simulink model "sim_environment_gcc"  (Simulink 8.6)
settings: Solver=VariableStepAuto  StartTime=0.0  StopTime=100  RelTol=1e-3
values from neighbouring files (symbols this model uses):
  controller_parameters = struct()    [sim_init.m]
  simulation_parameters = struct()    [sim_init.m]
  vehicle_parameters = struct()    [sim_init.m]
libraries: aerolibactuator x3
settings Model: Creator=cmasserafilho  LastModifiedBy=cmasserafilho
settings DataIOCC: LimitDataPoints=off  SaveFormat=Dataset  SignalLoggingSaveFormat=Dataset  ReturnWorkspaceOutputs=on
settings OptimizationCC: ExpressionDepthLimit=128
settings DebuggingCC: UnderspecifiedInitializationDetection=Simplified  MergeDetectMultiDrivingBlocksExec=error  SolverPrmCheckMsg=none  FcnCallInpInsideContextMsg=EnableAllAsError  StateNameClashWarn=none
settings HardwareCC: ProdBitPerPointer=64  ProdLargestAtomicFloat=Float  ProdIntDivRoundTo=Zero  ProdEndianess=LittleEndian  ProdWordSize=64  ProdHWDeviceType=Intel->x86-64 (Windows64)
settings GRTTargetCC: GeneratePreprocessorConditionals=Use local settings  CombineOutputUpdateFcns=on  GRTInterface=off
settings ConfigComp: CovModelRefEnable=off

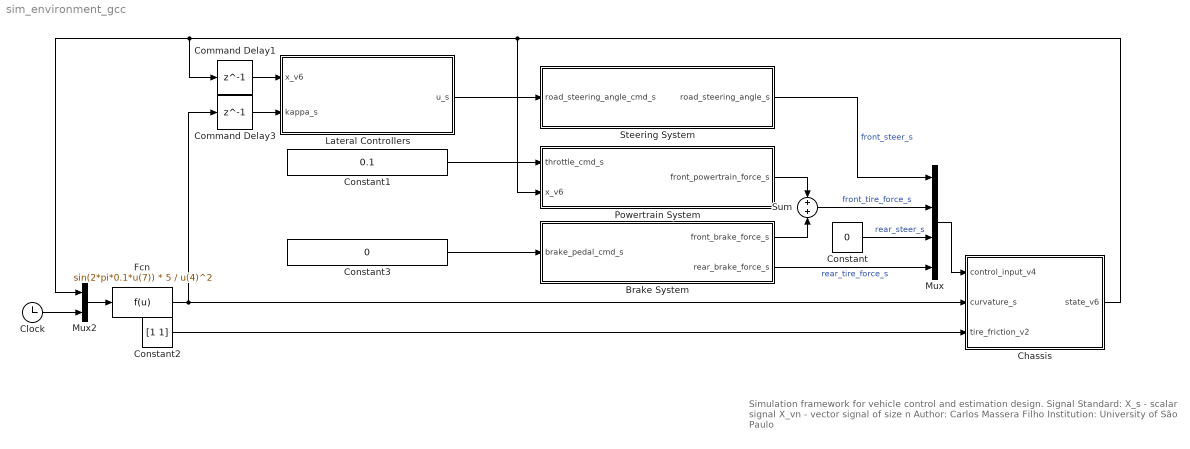
== system sim_environment_gcc ==
  note: Simulation framework for vehicle control and estimation design.
      |
      | Signal Standard:
      | X_s - scalar signal
      | X_vn - vector signal of size n
      |
      | Author: Carlos Massera Filho
      | Institution: University of São Paulo
  Brake System : Subsystem
  Chassis : Subsystem
  Clock : Clock
  Command Delay1 : Delay  DelayLength=1  InitialCondition=0  SampleTime=controller_parameters.Ts
  Command Delay3 : Delay  DelayLength=1  InitialCondition=0  SampleTime=controller_parameters.Ts
  Constant : Constant  Value=0
  Constant1 : Constant  Value=0.1  SampleTime=Inf
  Constant2 : Constant  Value=[1 1]
  Constant3 : Constant  Value=0
  Fcn : Fcn  Expr=sin(2*pi*0.1*u(7)) * 5 / u(4)^2
  Lateral Controllers : MATLAB Function  TreatAsAtomicUnit=on
  Mux : Mux
  Mux2 : Mux  Inputs=2
  Powertrain System : Subsystem
  Steering System : Subsystem
  Sum : Sum  Inputs=+|+
  wires:
  Chassis/1(state_v6) -> Command Delay1/1, Mux2/1, Powertrain System/2(x_v6)
  Mux/1 -> Chassis/1(control_input_v4)
  Constant/1 -> Mux/3  "rear_steer_s"
  Sum/1 -> Mux/2  "front_tire_force_s"
  Brake System/2(rear_brake_force_s) -> Mux/4  "rear_tire_force_s"
  Brake System/1(front_brake_force_s) -> Sum/2
  Powertrain System/1(front_powertrain_force_s) -> Sum/1
  Steering System/1("road_steering_angle_s ") -> Mux/1  "front_steer_s"
  Lateral Controllers/1(u_s) -> Steering System/1(road_steering_angle_cmd_s)
  Constant2/1 -> Chassis/3(tire_friction_v2)
  Command Delay1/1 -> Lateral Controllers/1(x_v6)
  Command Delay3/1 -> Lateral Controllers/2(kappa_s)
  Fcn/1 -> Command Delay3/1, Chassis/2(curvature_s)
  Mux2/1 -> Fcn/1
  Clock/1 -> Mux2/2
  Constant3/1 -> Brake System/1(brake_pedal_cmd_s)
  Constant1/1 -> Powertrain System/1(throttle_cmd_s)

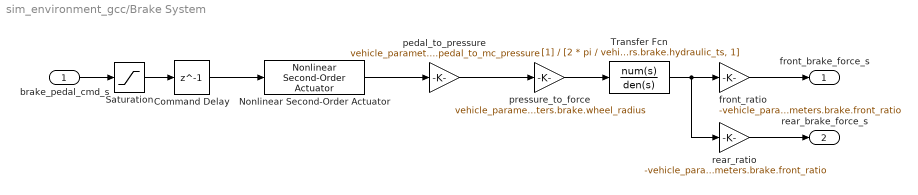
== system sim_environment_gcc/Brake System ==
  brake_pedal_cmd_s : Inport
  Command Delay : Delay  DelayLength=1  InitialCondition=0  SampleTime=vehicle_parameters.brake.delay
  Nonlinear Second-Order Actuator : aerolibactuator/Nonlinear Second-Order Actuator  wn_fin=2 * pi / vehicle_parameters.brake.actuator_tc  z_fin=1  fin_max=1  fin_min=0  fin_maxrate=vehicle_parameters.brake.rate_limit  fin_act_0=0  fin_act_vel=0
  Saturation : Saturate  UpperLimit=1  LowerLimit=0
  Transfer Fcn : TransferFcn  Denominator=[2 * pi / vehicle_parameters.brake.hydraulic_ts, 1]
  front_ratio : Gain  Gain=-vehicle_parameters.brake.front_ratio
  pedal_to_pressure : Gain  Gain=vehicle_parameters.brake.pedal_to_mc_pressure
  pressure_to_force : Gain  Gain=vehicle_parameters.brake.mc_pressure_to_torque / vehicle_parameters.brake.wheel_radius
  rear_ratio : Gain  Gain=-vehicle_parameters.brake.front_ratio
  front_brake_force_s : Outport
  rear_brake_force_s : Outport  Port=2
  wires:
  brake_pedal_cmd_s/1 -> Saturation/1
  front_ratio/1 -> front_brake_force_s/1
  rear_ratio/1 -> rear_brake_force_s/1
  Saturation/1 -> Command Delay/1
  Nonlinear Second-Order Actuator/1 -> pedal_to_pressure/1
  Command Delay/1 -> Nonlinear Second-Order Actuator/1
  pressure_to_force/1 -> Transfer Fcn/1
  Transfer Fcn/1 -> rear_ratio/1, front_ratio/1
  pedal_to_pressure/1 -> pressure_to_force/1

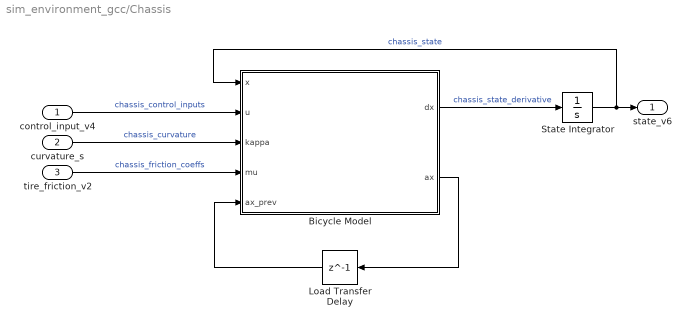
== system sim_environment_gcc/Chassis ==
  control_input_v4 : Inport
  curvature_s : Inport  Port=2
  tire_friction_v2 : Inport  Port=3
  Bicycle Model : MATLAB Function  TreatAsAtomicUnit=on
  Load Transfer Delay : Delay  DelayLength=1  InitialCondition=0  SampleTime=vehicle_parameters.uncertainty.load_transfer_Ts
  State Integrator : Integrator  InitialCondition=simulation_parameters.x0
  state_v6 : Outport
  wires:
  control_input_v4/1 -> Bicycle Model/2(u)  "chassis_control_inputs"
  State Integrator/1 -> state_v6/1, Bicycle Model/1(x)  "chassis_state"
  Load Transfer Delay/1 -> Bicycle Model/5(ax_prev)
  curvature_s/1 -> Bicycle Model/3(kappa)  "chassis_curvature"
  Bicycle Model/2(ax) -> Load Transfer Delay/1
  Bicycle Model/1(dx) -> State Integrator/1  "chassis_state_derivative"
  tire_friction_v2/1 -> Bicycle Model/4(mu)  "chassis_friction_coeffs"

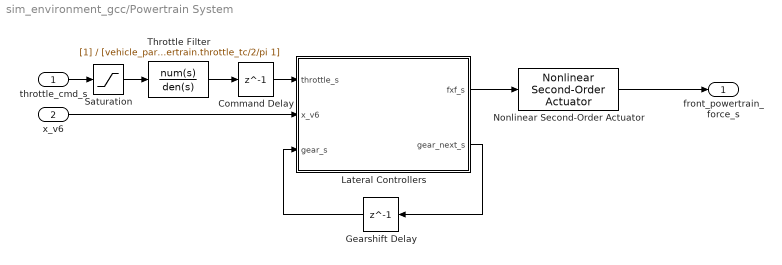
== system sim_environment_gcc/Powertrain System ==
  throttle_cmd_s : Inport
  x_v6 : Inport  Port=2
  Command Delay : Delay  DelayLength=1  InitialCondition=0  SampleTime=vehicle_parameters.powertrain.delay
  Gearshift Delay : Delay  DelayLength=1  InitialCondition=0  SampleTime=vehicle_parameters.powertrain.gear_shift_delay
  Lateral Controllers : MATLAB Function  TreatAsAtomicUnit=on
  Nonlinear Second-Order Actuator : aerolibactuator/Nonlinear Second-Order Actuator  wn_fin=2 * pi / vehicle_parameters.powertrain.engine_tc  z_fin=1  fin_max=Inf  fin_min=-Inf  fin_maxrate=Inf  fin_act_0=0  fin_act_vel=0
  Saturation : Saturate  UpperLimit=1  LowerLimit=0
  Throttle Filter : TransferFcn  Denominator=[vehicle_parameters.powertrain.throttle_tc/2/pi 1]
  front_powertrain_force_s : Outport
  wires:
  Lateral Controllers/1(fxf_s) -> Nonlinear Second-Order Actuator/1
  throttle_cmd_s/1 -> Saturation/1
  Throttle Filter/1 -> Command Delay/1
  Lateral Controllers/2(gear_next_s) -> Gearshift Delay/1
  Gearshift Delay/1 -> Lateral Controllers/3(gear_s)
  Nonlinear Second-Order Actuator/1 -> front_powertrain_force_s/1
  x_v6/1 -> Lateral Controllers/2(x_v6)
  Command Delay/1 -> Lateral Controllers/1(throttle_s)
  Saturation/1 -> Throttle Filter/1

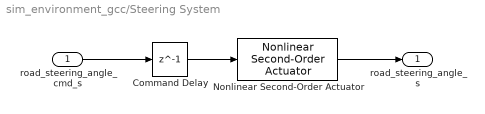
== system sim_environment_gcc/Steering System ==
  road_steering_angle_cmd_s : Inport
  Command Delay : Delay  DelayLength=1  InitialCondition=0  SampleTime=vehicle_parameters.steering.delay
  Nonlinear Second-Order Actuator : aerolibactuator/Nonlinear Second-Order Actuator  wn_fin=2 * pi / vehicle_parameters.steering.tc  z_fin=1  fin_max=vehicle_parameters.steering.angle_limit  fin_min=-vehicle_parameters.steering.angle_limit  fin_maxrate=vehicle_parameters.steering.rate_limit  fin_act_0=0  fin_act_vel=0
  "road_steering_angle_s " : Outport
  wires:
  road_steering_angle_cmd_s/1 -> Command Delay/1
  Command Delay/1 -> Nonlinear Second-Order Actuator/1
  Nonlinear Second-Order Actuator/1 -> "road_steering_angle_s "/1

== matlab function Lateral Controllers ==
  data: x_v6 input double; u_s output double; kappa_s input double; controller parameter double
function u_s = gcc_control_wrapper(x_v6, kappa_s, controller)

    u_s = gcc_control(x_v6, kappa_s, controller);
    
end

== matlab function Chassis/Bicycle Model ==
  data: x input double; u input double size=4; dx output double; kappa input double; mu input double; ax_prev input double; vehicle_parameters parameter double; ax output double
function [dx, ax] = bicycle_model_wrapper(x, u, kappa, mu, ax_prev, vehicle_parameters)

    [dx, ax] = nonliear_bicycle_model(x, u, kappa, mu, ax_prev, vehicle_parameters);
    
end

== matlab function Powertrain System/Lateral Controllers ==
  data: throttle_s input double; x_v6 input double; gear_s input double; fxf_s output double; vehicle_parameters parameter double; gear_next_s output double
function [fxf_s, gear_next_s] = powertrain_model_wrapper(throttle_s, x_v6, gear_s, vehicle_parameters)

    [fxf_s, gear_next_s] = powertrain_model(throttle_s, x_v6, gear_s, vehicle_parameters.powertrain);
    
end
